simulink model "Taller5_TDCM"  (R2024a)
settings: Solver=VariableStepAuto  StartTime=0.0  StopTime=0.050  RelTol=1e-3
values from neighbouring files (symbols this model uses):
  den = [1 R/L 1/(L*C)]    [Taller5_TDCM.m]
  num = 1/(L*C)    (= 45454.5454545)    [Taller5_TDCM.m]
libraries: slpidlib x1
settings Model: Creator=emili  LastModifiedBy=emili

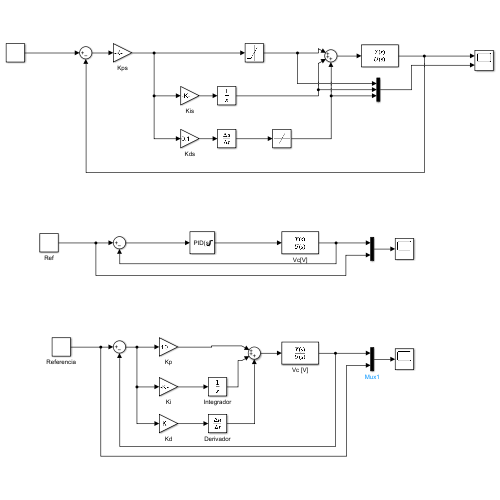
[thumbnail: Simulink's stored preview of the top-level diagram]
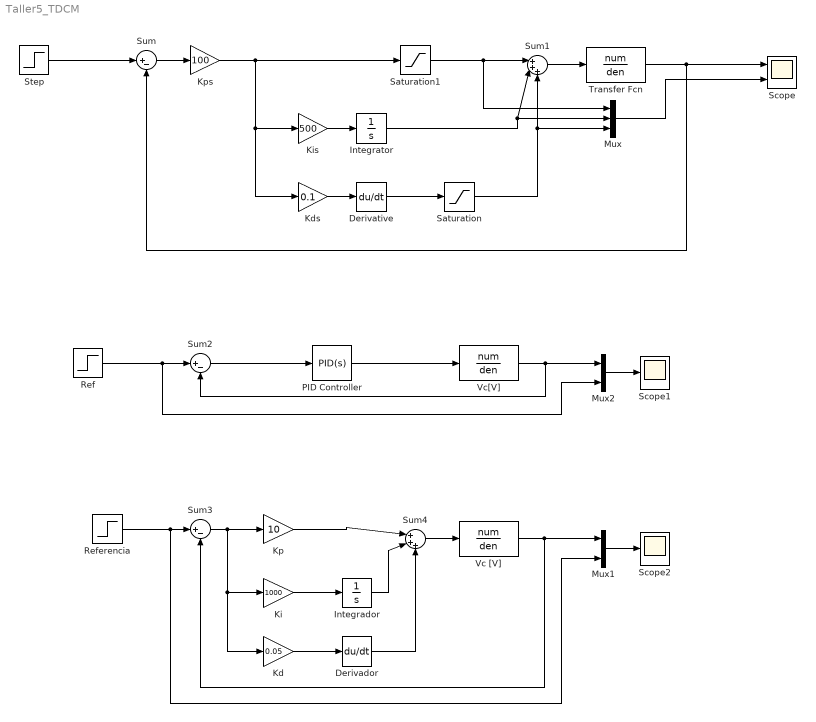
== system Taller5_TDCM ==
  Derivador : Derivative
  Derivative : Derivative
  Integrador : Integrator
  Integrator : Integrator
  Kd : Gain  Gain=0.05
  Kds : Gain  Gain=0.1
  Ki : Gain  Gain=1000
  Kis : Gain  Gain=500
  Kp : Gain  Gain=10
  Kps : Gain  Gain=100
  Mux : Mux  Inputs=3
  Mux1 : Mux  Inputs=2
  Mux2 : Mux  Inputs=2
  PID Controller : slpidlib/PID Controller  Controller=PID  Form=Parallel  TimeDomain=Continuous-time  UseExternalTs=off  SampleTime=-1  IntegratorMethod=Forward Euler  FilterMethod=Forward Euler  ControllerParametersSource=internal  P=8.27881880837983  I=614.585464581946  UseKiTs=off  D=0.0195243747538086  UseExternalDerivativeSource=off  N=10597.7305256217  UseFilter=on  TunerSelectOption=Transfer Function Based (PID Tuner App)  InitialConditionSource=internal  InitialConditionForIntegrator=0  InitialConditionForFilter=0  DifferentiatorICPrevScaledInput=0  ExternalReset=none  TrackingMode=off  Kt=1  LimitOutput=on  SatLimitsSource=internal  UpperSaturationLimit=15  LowerSaturationLimit=-15  LinearizeAsGain=on  AntiWindupMode=none  Kb=1  LimitIntegrator=on  UpperIntegratorSaturationLimit=15  LowerIntegratorSaturationLimit=-15  POutMin=[]  POutMax=[]  IOutMin=[]  IOutMax=[]  DOutMin=[]  DOutMax=[]  NOutMin=[]  NOutMax=[]  SumOutMin=[]  SumOutMax=[]  SaturationOutMin=[]  SaturationOutMax=[]  PParamMin=[]  PParamMax=[]  IParamMin=[]  IParamMax=[]  DParamMin=[]  DParamMax=[]  NParamMin=[]  NParamMax=[]  KbParamMin=[]  KbParamMax=[]  KtParamMin=[]  KtParamMax=[]  KbOutMin=[]  KbOutMax=[]  KtOutMin=[]  KtOutMax=[]  IntegratorOutMin=[]  IntegratorOutMax=[]  FilterOutMin=[]  FilterOutMax=[]  SumI1OutMin=[]  SumI1OutMax=[]  SumI2OutMin=[]  SumI2OutMax=[]  SumI3OutMin=[]  SumI3OutMax=[]  SumI4OutMin=[]  SumI4OutMax=[]  SumDOutMin=[]  SumDOutMax=[]  DifferentiatorOutMin=[]  DifferentiatorOutMax=[]  FilterDiffOutCoefMin=[]  FilterDiffOutCoefMax=[]  ReciprocalOutMin=[]  ReciprocalOutMax=[]  SumDenOutMin=[]  SumDenOutMax=[]  SumNumOutMin=[]  SumNumOutMax=[]  DivideOutMin=[]  DivideOutMax=[]  UdiffTsProdOutMin=[]  UdiffTsProdOutMax=[]  NTsProdOutMin=[]  NTsProdOutMax=[]  UintegralTsProdOutMin=[]  UintegralTsProdOutMax=[]  UngainTsProdOutMin=[]  UngainTsProdOutMax=[]  ClampingZeroOutDataTypeStr=Inherit: Inherit via back propagation  ClampingZeroOutMin=[]  ClampingZeroOutMax=[]  FilterDenConstantOutDataTypeStr=Inherit: Inherit via back propagation  FilterDenConstantOutMin=[]  FilterDenConstantOutMax=[]  PCopyOutDataTypeStr=Inherit: Inherit via back propagation  PCopyOutMin=[]  PCopyOutMax=[]  NCopyOutDataTypeStr=Inherit: Inherit via back propagation  NCopyOutMin=[]  NCopyOutMax=[]  IntegratorContinuousStateAttributes=''  IntegratorStateMustResolveToSignalObject=off  IntegratorRTWStateStorageClass=Auto  FilterContinuousStateAttributes=''  FilterStateMustResolveToSignalObject=off  FilterRTWStateStorageClass=Auto  ParallelPVariant=InternalParameters  IdealPVariant=Disabled  IVariant=InternalParameters  DVariant=InternalParameters  IntegratorVariant=Continuous  SatVariant=Enabled  AWVariant=Passthrough  PCopyVariant=Disabled  TRVariant=Disabled  FdbkBlocksVariant=Forward  IdealPFdbkVariant=Disabled  SatFdbkVariant=Disabled  DerivativeFilterVariant=ContFilter  NVariant=InternalParameters  NCopyVariant=Disabled  FilterICVariant=InternalICsFilter  IntegratorICVariant=InternalICs  ExternalResetVariant=Disabled  TRSumVariant=Passthrough  SumFdbkVariant=Disabled  SumVariant=Sum_PID  TsampFilterVariant=InternalTs  TsampNgainVariant=Passthrough  TsampIntegralVariant=Disabled_SignalSpec  ExternalSaturationOutDataTypeStr=Inherit: Same as second input  DerivativeSourceVariant=ErrorSignal
  Ref : Step  Time=0.01  After=5  SampleTime=0
  Referencia : Step  Time=0.01  After=5  SampleTime=0
  Saturation : Saturate  UpperLimit=15  LowerLimit=-15  ZeroCross=off
  Saturation1 : Saturate  UpperLimit=15  LowerLimit=-15  ZeroCross=off
  Scope : Scope  NumInputPorts=2
  Scope1 : Scope
  Scope2 : Scope
  Step : Step  Time=0.01  SampleTime=0
  Sum : Sum  Inputs=|+-
  Sum1 : Sum  Inputs=|+++
  Sum2 : Sum  Inputs=|+-
  Sum3 : Sum  Inputs=|+-
  Sum4 : Sum  Inputs=|+++
  Transfer Fcn : TransferFcn  Numerator=num  Denominator=den
  Vc [V] : TransferFcn  Numerator=num  Denominator=den
  Vc[V] : TransferFcn  Numerator=num  Denominator=den
  wires:
  Step/1 -> Sum/1
  Sum/1 -> Kps/1
  Transfer Fcn/1 -> Sum/2, Scope/1
  Sum1/1 -> Transfer Fcn/1
  Kis/1 -> Integrator/1
  Kds/1 -> Derivative/1
  Derivative/1 -> Saturation/1
  Mux/1 -> Scope/2
  Saturation/1 -> Mux/3, Sum1/3
  Saturation1/1 -> Mux/1, Sum1/1
  Integrator/1 -> Mux/2, Sum1/2
  Kps/1 -> Saturation1/1, Kds/1, Kis/1
  Ref/1 -> Mux2/2, Sum2/1
  Vc[V]/1 -> Mux2/1, Sum2/2
  Sum2/1 -> PID Controller/1
  PID Controller/1 -> Vc[V]/1
  Referencia/1 -> Mux1/2, Sum3/1
  Vc [V]/1 -> Mux1/1, Sum3/2
  Mux1/1 -> Scope2/1
  Sum3/1 -> Kd/1, Ki/1, Kp/1
  Kp/1 -> Sum4/1
  Sum4/1 -> Vc [V]/1
  Integrador/1 -> Sum4/2
  Ki/1 -> Integrador/1
  Kd/1 -> Derivador/1
  Derivador/1 -> Sum4/3
  Mux2/1 -> Scope1/1
